simulink model "warplab_pkt_proc"  (Simulink 7.8)
settings: Solver=ode45  StartTime=0.0  StopTime=10.0  RelTol=1e-3
undefined symbols (not defined in the file): gcbh, xlBlockLoadCallback, xlGetNormalizedPeriod
libraries: xbsIndex_r4 x230, xbsEDKLib_r4 x1
(part 4 of 4)

== system warplab_pkt_proc/Pkt Comp/Word Comp 0/Byte Comp 1/Equal ==
  D : Inport
  BT : Inport  Port=2
  Relational : xbsIndex_r4/Relational  mode=a=b  en=off  latency=0  dbl_ovrd=off  block_type=relational
  R : Outport
  wires:
  Relational/1 -> R/1
  BT/1 -> Relational/2
  D/1 -> Relational/1

== system warplab_pkt_proc/Pkt Comp/Word Comp 0/Byte Comp 1/Not Equal ==
  D : Inport
  BT : Inport  Port=2
  Relational : xbsIndex_r4/Relational  mode=a!=b  en=off  latency=0  dbl_ovrd=off  block_type=relational
  R : Outport
  wires:
  D/1 -> Relational/1
  BT/1 -> Relational/2
  Relational/1 -> R/1

== system warplab_pkt_proc/Pkt Comp/Word Comp 0/Byte Comp 2/Any of AND ==
  D : Inport
  T : Inport  Port=2
  Constant3 : xbsIndex_r4/Constant  const=0  gui_display_data_type=Fixed-point  arith_type=Unsigned  n_bits=8  bin_pt=0  preci_type=Single  exp_width=8  frac_width=24  explicit_period=off  period=1  equ=P=C  opselect=C  inp2=PCIN>>17  opr=+  inp1=P  carry=CIN  dbl_ovrd=off  block_type=constant
  Logical : xbsIndex_r4/Logical  logical_function=AND  inputs=2  en=off  latency=0  precision=Full  arith_type=Unsigned  n_bits=16  bin_pt=0  align_bp=on  dbl_ovrd=off  block_type=logical
  Relational1 : xbsIndex_r4/Relational  mode=a!=b  en=off  latency=0  dbl_ovrd=off  block_type=relational
  R : Outport
  wires:
  Constant3/1 -> Relational1/1
  Logical/1 -> Relational1/2
  D/1 -> Logical/1
  T/1 -> Logical/2
  Relational1/1 -> R/1

== system warplab_pkt_proc/Pkt Comp/Word Comp 0/Byte Comp 2/Equal ==
  D : Inport
  BT : Inport  Port=2
  Relational : xbsIndex_r4/Relational  mode=a=b  en=off  latency=0  dbl_ovrd=off  block_type=relational
  R : Outport
  wires:
  D/1 -> Relational/1
  BT/1 -> Relational/2
  Relational/1 -> R/1

== system warplab_pkt_proc/Pkt Comp/Word Comp 0/Byte Comp 2/Not Equal ==
  D : Inport
  BT : Inport  Port=2
  Relational : xbsIndex_r4/Relational  mode=a!=b  en=off  latency=0  dbl_ovrd=off  block_type=relational
  R : Outport
  wires:
  Relational/1 -> R/1
  BT/1 -> Relational/2
  D/1 -> Relational/1

== system warplab_pkt_proc/Pkt Comp/Word Comp 0/Byte Comp 3/Any of AND ==
  D : Inport
  T : Inport  Port=2
  Constant3 : xbsIndex_r4/Constant  const=0  gui_display_data_type=Fixed-point  arith_type=Unsigned  n_bits=8  bin_pt=0  preci_type=Single  exp_width=8  frac_width=24  explicit_period=off  period=1  equ=P=C  opselect=C  inp2=PCIN>>17  opr=+  inp1=P  carry=CIN  dbl_ovrd=off  block_type=constant
  Logical : xbsIndex_r4/Logical  logical_function=AND  inputs=2  en=off  latency=0  precision=Full  arith_type=Unsigned  n_bits=16  bin_pt=0  align_bp=on  dbl_ovrd=off  block_type=logical
  Relational1 : xbsIndex_r4/Relational  mode=a!=b  en=off  latency=0  dbl_ovrd=off  block_type=relational
  R : Outport
  wires:
  Relational1/1 -> R/1
  T/1 -> Logical/2
  D/1 -> Logical/1
  Logical/1 -> Relational1/2
  Constant3/1 -> Relational1/1

== system warplab_pkt_proc/Pkt Comp/Word Comp 0/Byte Comp 3/Equal ==
  D : Inport
  BT : Inport  Port=2
  Relational : xbsIndex_r4/Relational  mode=a=b  en=off  latency=0  dbl_ovrd=off  block_type=relational
  R : Outport
  wires:
  Relational/1 -> R/1
  BT/1 -> Relational/2
  D/1 -> Relational/1

== system warplab_pkt_proc/Pkt Comp/Word Comp 0/Byte Comp 3/Not Equal ==
  D : Inport
  BT : Inport  Port=2
  Relational : xbsIndex_r4/Relational  mode=a!=b  en=off  latency=0  dbl_ovrd=off  block_type=relational
  R : Outport
  wires:
  D/1 -> Relational/1
  BT/1 -> Relational/2
  Relational/1 -> R/1

== system warplab_pkt_proc/Pkt Comp/Word Comp 1/Byte Comp 0/Any of AND ==
  D : Inport
  T : Inport  Port=2
  Constant3 : xbsIndex_r4/Constant  const=0  gui_display_data_type=Fixed-point  arith_type=Unsigned  n_bits=8  bin_pt=0  preci_type=Single  exp_width=8  frac_width=24  explicit_period=off  period=1  equ=P=C  opselect=C  inp2=PCIN>>17  opr=+  inp1=P  carry=CIN  dbl_ovrd=off  block_type=constant
  Logical : xbsIndex_r4/Logical  logical_function=AND  inputs=2  en=off  latency=0  precision=Full  arith_type=Unsigned  n_bits=16  bin_pt=0  align_bp=on  dbl_ovrd=off  block_type=logical
  Relational1 : xbsIndex_r4/Relational  mode=a!=b  en=off  latency=0  dbl_ovrd=off  block_type=relational
  R : Outport
  wires:
  Relational1/1 -> R/1
  T/1 -> Logical/2
  D/1 -> Logical/1
  Logical/1 -> Relational1/2
  Constant3/1 -> Relational1/1

== system warplab_pkt_proc/Pkt Comp/Word Comp 1/Byte Comp 0/Equal ==
  D : Inport
  BT : Inport  Port=2
  Relational : xbsIndex_r4/Relational  mode=a=b  en=off  latency=0  dbl_ovrd=off  block_type=relational
  R : Outport
  wires:
  Relational/1 -> R/1
  BT/1 -> Relational/2
  D/1 -> Relational/1

== system warplab_pkt_proc/Pkt Comp/Word Comp 1/Byte Comp 0/Not Equal ==
  D : Inport
  BT : Inport  Port=2
  Relational : xbsIndex_r4/Relational  mode=a!=b  en=off  latency=0  dbl_ovrd=off  block_type=relational
  R : Outport
  wires:
  D/1 -> Relational/1
  BT/1 -> Relational/2
  Relational/1 -> R/1

== system warplab_pkt_proc/Pkt Comp/Word Comp 1/Byte Comp 1/Any of AND ==
  D : Inport
  T : Inport  Port=2
  Constant3 : xbsIndex_r4/Constant  const=0  gui_display_data_type=Fixed-point  arith_type=Unsigned  n_bits=8  bin_pt=0  preci_type=Single  exp_width=8  frac_width=24  explicit_period=off  period=1  equ=P=C  opselect=C  inp2=PCIN>>17  opr=+  inp1=P  carry=CIN  dbl_ovrd=off  block_type=constant
  Logical : xbsIndex_r4/Logical  logical_function=AND  inputs=2  en=off  latency=0  precision=Full  arith_type=Unsigned  n_bits=16  bin_pt=0  align_bp=on  dbl_ovrd=off  block_type=logical
  Relational1 : xbsIndex_r4/Relational  mode=a!=b  en=off  latency=0  dbl_ovrd=off  block_type=relational
  R : Outport
  wires:
  Constant3/1 -> Relational1/1
  Logical/1 -> Relational1/2
  D/1 -> Logical/1
  T/1 -> Logical/2
  Relational1/1 -> R/1

== system warplab_pkt_proc/Pkt Comp/Word Comp 1/Byte Comp 1/Equal ==
  D : Inport
  BT : Inport  Port=2
  Relational : xbsIndex_r4/Relational  mode=a=b  en=off  latency=0  dbl_ovrd=off  block_type=relational
  R : Outport
  wires:
  D/1 -> Relational/1
  BT/1 -> Relational/2
  Relational/1 -> R/1

== system warplab_pkt_proc/Pkt Comp/Word Comp 1/Byte Comp 1/Not Equal ==
  D : Inport
  BT : Inport  Port=2
  Relational : xbsIndex_r4/Relational  mode=a!=b  en=off  latency=0  dbl_ovrd=off  block_type=relational
  R : Outport
  wires:
  Relational/1 -> R/1
  BT/1 -> Relational/2
  D/1 -> Relational/1

== system warplab_pkt_proc/Pkt Comp/Word Comp 1/Byte Comp 2/Any of AND ==
  D : Inport
  T : Inport  Port=2
  Constant3 : xbsIndex_r4/Constant  const=0  gui_display_data_type=Fixed-point  arith_type=Unsigned  n_bits=8  bin_pt=0  preci_type=Single  exp_width=8  frac_width=24  explicit_period=off  period=1  equ=P=C  opselect=C  inp2=PCIN>>17  opr=+  inp1=P  carry=CIN  dbl_ovrd=off  block_type=constant
  Logical : xbsIndex_r4/Logical  logical_function=AND  inputs=2  en=off  latency=0  precision=Full  arith_type=Unsigned  n_bits=16  bin_pt=0  align_bp=on  dbl_ovrd=off  block_type=logical
  Relational1 : xbsIndex_r4/Relational  mode=a!=b  en=off  latency=0  dbl_ovrd=off  block_type=relational
  R : Outport
  wires:
  Relational1/1 -> R/1
  T/1 -> Logical/2
  D/1 -> Logical/1
  Logical/1 -> Relational1/2
  Constant3/1 -> Relational1/1

== system warplab_pkt_proc/Pkt Comp/Word Comp 1/Byte Comp 2/Equal ==
  D : Inport
  BT : Inport  Port=2
  Relational : xbsIndex_r4/Relational  mode=a=b  en=off  latency=0  dbl_ovrd=off  block_type=relational
  R : Outport
  wires:
  Relational/1 -> R/1
  BT/1 -> Relational/2
  D/1 -> Relational/1

== system warplab_pkt_proc/Pkt Comp/Word Comp 1/Byte Comp 2/Not Equal ==
  D : Inport
  BT : Inport  Port=2
  Relational : xbsIndex_r4/Relational  mode=a!=b  en=off  latency=0  dbl_ovrd=off  block_type=relational
  R : Outport
  wires:
  D/1 -> Relational/1
  BT/1 -> Relational/2
  Relational/1 -> R/1

== system warplab_pkt_proc/Pkt Comp/Word Comp 1/Byte Comp 3/Any of AND ==
  D : Inport
  T : Inport  Port=2
  Constant3 : xbsIndex_r4/Constant  const=0  gui_display_data_type=Fixed-point  arith_type=Unsigned  n_bits=8  bin_pt=0  preci_type=Single  exp_width=8  frac_width=24  explicit_period=off  period=1  equ=P=C  opselect=C  inp2=PCIN>>17  opr=+  inp1=P  carry=CIN  dbl_ovrd=off  block_type=constant
  Logical : xbsIndex_r4/Logical  logical_function=AND  inputs=2  en=off  latency=0  precision=Full  arith_type=Unsigned  n_bits=16  bin_pt=0  align_bp=on  dbl_ovrd=off  block_type=logical
  Relational1 : xbsIndex_r4/Relational  mode=a!=b  en=off  latency=0  dbl_ovrd=off  block_type=relational
  R : Outport
  wires:
  Constant3/1 -> Relational1/1
  Logical/1 -> Relational1/2
  D/1 -> Logical/1
  T/1 -> Logical/2
  Relational1/1 -> R/1

== system warplab_pkt_proc/Pkt Comp/Word Comp 1/Byte Comp 3/Equal ==
  D : Inport
  BT : Inport  Port=2
  Relational : xbsIndex_r4/Relational  mode=a=b  en=off  latency=0  dbl_ovrd=off  block_type=relational
  R : Outport
  wires:
  D/1 -> Relational/1
  BT/1 -> Relational/2
  Relational/1 -> R/1

== system warplab_pkt_proc/Pkt Comp/Word Comp 1/Byte Comp 3/Not Equal ==
  D : Inport
  BT : Inport  Port=2
  Relational : xbsIndex_r4/Relational  mode=a!=b  en=off  latency=0  dbl_ovrd=off  block_type=relational
  R : Outport
  wires:
  Relational/1 -> R/1
  BT/1 -> Relational/2
  D/1 -> Relational/1
